simulink model "Res_8"  (R2018b)
settings: Solver=ode4  StartTime=0.0  StopTime=1.5  FixedStep=0.0001  RelTol=1e-3
settings Model: Creator=makha  LastModifiedBy=makha

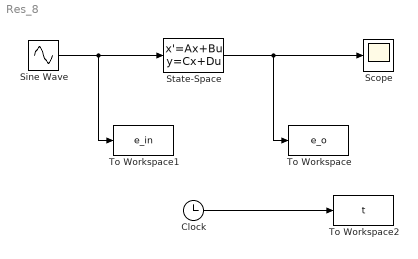
== system Res_8 ==
  Clock : Clock
  Scope : Scope
  Sine Wave : Sin  Amplitude=0.5  Frequency=10  SampleTime=0.0001
  State-Space : StateSpace  A=[-20 -100; 25 -62.5]  B=[100; 62.5]  C=[0 1]  D=0  InitialCondition=[0; 0.25]
  To Workspace : ToWorkspace  VariableName=e_o  SampleTime=-1
  To Workspace1 : ToWorkspace  VariableName=e_in  SampleTime=-1
  To Workspace2 : ToWorkspace  VariableName=t  SampleTime=-1
  wires:
  Sine Wave/1 -> To Workspace1/1, State-Space/1
  State-Space/1 -> To Workspace/1, Scope/1
  Clock/1 -> To Workspace2/1
